simulink model "fuzzyPDdeo1"  (R2025b)
settings: Solver=VariableStepAuto  StartTime=0.0  StopTime=300  RelTol=1e-3
libraries: fuzblock x1

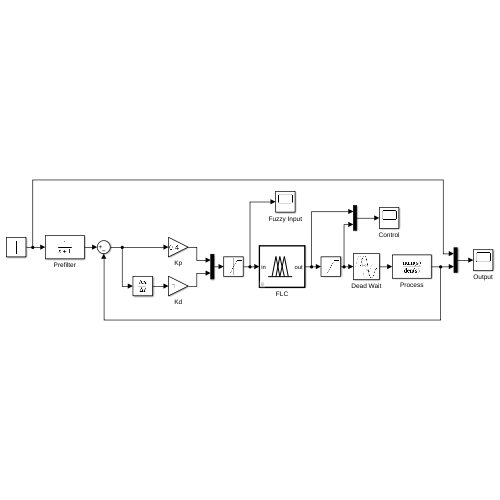
[thumbnail: Simulink's stored preview of the top-level diagram]
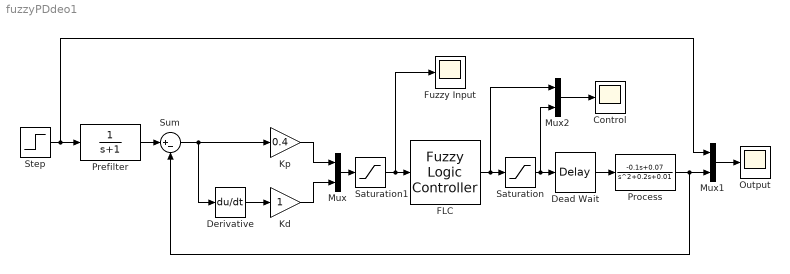
== system fuzzyPDdeo1 ==
  Control : Scope
      settings: ActiveDisplayYMinimum=-2.1941211043383504  ActiveDisplayYMaximum=2.4103369668835777
  Dead Wait : TransportDelay  DelayTime=3
  Derivative : Derivative
  FLC : fuzblock/Fuzzy Logic  Controller  FIS='Copy_of_fuzzyPDmodel.fis'  OutputSampleNumber=101  DataType=double  UseLookupTable=off  NumBreakpoints=10  FuzzifiedInputs=off  RuleFiringStrengths=off  RuleOutputs=off  AggregatedOutputs=off  SimulateUsing=Interpreted execution  OutOfRangeInputValueMessage=warning  NoRuleFiredMessage=warning  EmptyOutputFuzzySetMessage=warning
  Fuzzy Input : Scope
      settings: ActiveDisplayYMinimum=-1.9597839163902746  ActiveDisplayYMaximum=3.6369636470429221  DataLoggingVariableName=ScopeData2
  Kd : Gain
  Kp : Gain  Gain=0.4
  Mux : Mux  Inputs=2
  Mux1 : Mux  Inputs=2
  Mux2 : Mux  Inputs=2
  Output : Scope
      settings: ActiveDisplayYMinimum=-2.5147921249307874  ActiveDisplayYMaximum=2.3198888498522372
  Prefilter : TransferFcn  Denominator=[1 1]
  Process : TransferFcn  Numerator=[-0.1 0.07]  Denominator=[1 0.2 0.01]
  Saturation : Saturate  UpperLimit=1.0  LowerLimit=-1.0
  Saturation1 : Saturate  UpperLimit=1.0  LowerLimit=-1.0
  Step : Step  Time=3  Before=-2.0  After=2.0  SampleTime=0
  Sum : Sum  Inputs=|+-
  wires:
  Sum/1 -> Kp/1, Derivative/1
  Kp/1 -> Mux/1
  Kd/1 -> Mux/2
  Derivative/1 -> Kd/1
  Process/1 -> Sum/2, Mux1/2
  Dead Wait/1 -> Process/1
  FLC/1 -> Mux2/1, Saturation/1
  Saturation/1 -> Mux2/2, Dead Wait/1
  Step/1 -> Prefilter/1, Mux1/1
  Prefilter/1 -> Sum/1
  Mux1/1 -> Output/1
  Mux2/1 -> Control/1
  Saturation1/1 -> Fuzzy Input/1, FLC/1
  Mux/1 -> Saturation1/1
